simulink model "SimulinkSampleMotorWheelMode_R2017a"  (R2019a)
settings: Solver=VariableStepAuto  StartTime=0.0  StopTime=10.0  RelTol=1e-3
libraries: instrumentlib x3
settings Model: Creator=go_71  LastModifiedBy=Eureka Dynamics
settings DebuggingCC: UnconnectedInputMsg=none  UnconnectedOutputMsg=none  UnconnectedLineMsg=none  ArithmeticOperatorsInVariantConditions=warning
settings ModelReferenceCC: EnableRefExpFcnMdlSchedulingChecks=off
settings RTWCC: Description=Generic Real-Time Target
settings CodeAppCC: StateflowObjectComments=on

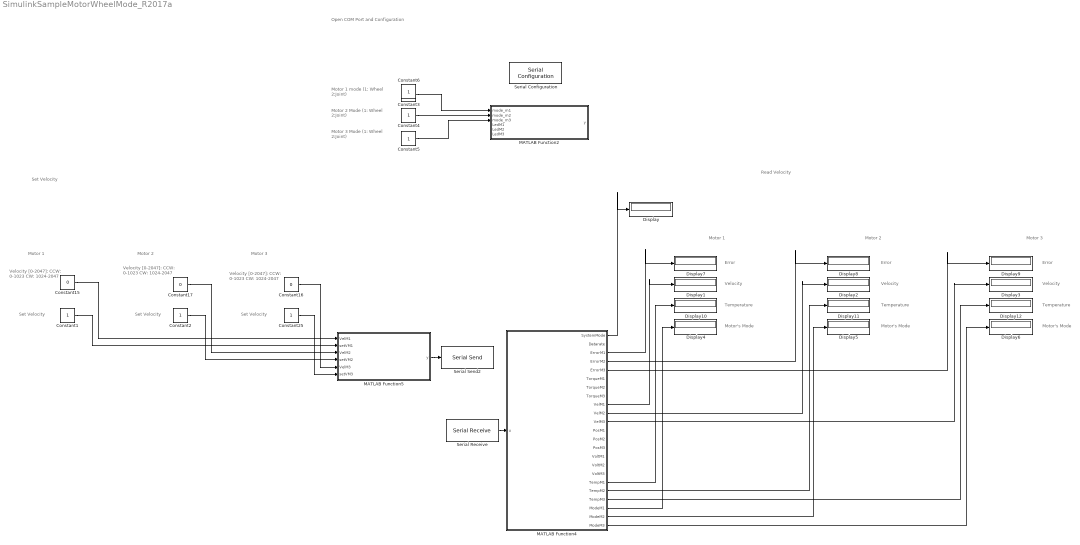
== system SimulinkSampleMotorWheelMode_R2017a ==
  note: Open COM Port and Configuration
  note: Motor's Mode
  note: Motor 3
  note: Temperature
  note: Error
  note: Temperature
  note: Error
  note: Velocity
  note: Velocity
  note: Motor's Mode
  note: Motor's Mode
  note: Error
  note: Temperature
  note: Velocity
  note: Motor 1
  note: Motor 2
  note: Motor 1 mode
      | (1: Wheel 2:Joint)
  note: Motor 2 Mode
      | (1: Wheel 2:Joint)
  note: Motor 3 Mode
      | (1: Wheel 2:Joint)
  note: Motor 1
  note: Motor 2
  note: Motor 3
  note: Read Velocity
  note: Set Velocity
  note: Velocity
      | [0-2047]:
      | CCW: 0-1023
      | CW: 1024-2047
  note: Set Velocity
  note: Set Velocity
  note: Velocity
      | [0-2047]:
      | CCW: 0-1023
      | CW: 1024-2047
  note: Set Velocity
  note: Velocity
      | [0-2047]:
      | CCW: 0-1023
      | CW: 1024-2047
  Constant{1..6,25} (7 alike) : Constant  SampleTime=1
  Constant15 : Constant  Value=0  SampleTime=1
  Constant16 : Constant  Value=0  SampleTime=1
  Constant17 : Constant  Value=0  SampleTime=1
  Display{,1..12} (13 alike) : Display
  MATLAB Function2 : MATLAB Function  Priority=1  TreatAsAtomicUnit=on  SystemSampleTime=1
  MATLAB Function4 : MATLAB Function  Priority=3  TreatAsAtomicUnit=on
  MATLAB Function5 : MATLAB Function  Priority=2  TreatAsAtomicUnit=on
  Serial Configuration : instrumentlib/Serial Configuration  Priority=-200000  ComPortMenu=<Please select a port...>  ComPort=<Please select a port...>  BaudRate=9600  DataBits=8  Parity=none  StopBits=1  FlowControl=none  Timeout=10  ByteOrder=LittleEndian
  Serial Receive : instrumentlib/Serial Receive  ComPortMenu=<Please select a port...>  ComPort=<Please select a port...>  DataSize="[32   1]"  DataType=uint8  EnableBlockingMode=on  ActionDataUnavailable=Output last received value  CustomValue=0  SampleTime=0.01
  Serial Send2 : instrumentlib/Serial Send  ComPortMenu=<Please select a port...>  ComPort=<Please select a port...>  Terminator=<none>  EnableBlockingMode=on
  wires:
  Constant3/1 -> MATLAB Function2/1(mode_m1)
  Constant5/1 -> MATLAB Function2/3(mode_m3)
  Constant25/1 -> MATLAB Function5/6(setVM3)
  Constant4/1 -> MATLAB Function2/2(mode_m2)
  Constant1/1 -> MATLAB Function5/2(setVM1)
  Constant2/1 -> MATLAB Function5/4(setVM2)
  Constant15/1 -> MATLAB Function5/1(VelM1)
  Constant17/1 -> MATLAB Function5/3(VelM2)
  Constant16/1 -> MATLAB Function5/5(VelM3)
  MATLAB Function4/22(ModeM2) -> Display5/1
  MATLAB Function4/21(ModeM1) -> Display4/1
  MATLAB Function4/20(TempM3) -> Display12/1
  MATLAB Function4/4(ErrorM2) -> Display8/1
  MATLAB Function4/19(TempM2) -> Display11/1
  MATLAB Function4/3(ErrorM1) -> Display7/1
  MATLAB Function4/1(SystemMode) -> Display/1
  Serial Receive/1 -> MATLAB Function4/1(u)
  MATLAB Function4/18(TempM1) -> Display10/1
  MATLAB Function4/5(ErrorM3) -> Display9/1
  MATLAB Function4/23(ModeM3) -> Display6/1
  MATLAB Function4/9(VelM1) -> Display1/1
  MATLAB Function4/10(VelM2) -> Display2/1
  MATLAB Function4/11(VelM3) -> Display3/1
  MATLAB Function5/1(y) -> Serial Send2/1

== matlab function SimulinkSampleMotorWheelMode_R2017a/MATLAB Function2 ==
  data: y output; mode_m1 input; mode_m2 input; mode_m3 input; LedM1 input; LedM2 input; LedM3 input
function y  = setMotorsConfiguration(mode_m1,mode_m2,mode_m3,LedM1,LedM2,LedM3)
% Motor Configuration Packet

% mode_m1=1 -> Wheel
% mode_m1=2 -> Joint

s.init          = 122;
s.mode          = 3;      % 3=motor configuration
s.set_mode_m1   = 48 ;    % 48 = char '0' 49 = char '1'
s.set_mode_m2   = 48 ;    % 48 = char '0' 49 = char '1'
s.set_mode_m3   = 48 ;    % 48 = char '0' 49 = char '1'
s.mode_m1       = 49 ;  %49 = char '1' Wheel   50 = char '2' Joint
s.mode_m2       = 49 ;  %49 = char '1' Wheel   50 = char '2' Joint
s.mode_m3       = 49 ;  %49 = char '1' Wheel   50 = char '2' Joint

if mode_m1~=0
    s.set_mode_m1 = 49 ;  
    if mode_m1==1 %Mode Wheel
        s.mode_m1 = 49 ;
    elseif mode_m1==2  
        s.mode_m1 = 50 ;  
    end
end

if mode_m2~=0
    s.set_mode_m2 = 49 ;   
    if mode_m2==1 % Mode Wheel
        s.mode_m2 = 49 ; 
    elseif mode_m2==2  
        s.mode_m2 = 50 ;
    end
end

if mode_m3~=0
    s.set_mode_m3 = 49 ; 
    if mode_m3 == 1 % Mode Wheel
        s.mode_m3 = 49 ; 
    elseif mode_m3==2  
        s.mode_m3 = 50 ;
    end
end


s.set_id_m1 = 0 ;
s.set_id_m2 = 0 ;
s.set_id_m3 = 0 ;

s.id_m1 = 0;
s.id_m2 = 0;
s.id_m3 = 0;

LEDM1 = 48;
if LedM1 ==1
    LEDM1 =49;
end

LEDM2 = 48;
if LedM2 ==1
    LEDM2 =49;
end

LEDM3 = 48;
if LedM3 ==1
    LEDM3 =49;
end

s.turnon_led_m1 = LEDM1;  %48:0  49:1
s.turnon_led_m2 = LEDM2;
s.turnon_led_m3 = LEDM3;
s.not_used17 = 0;
s.not_used18 = 0;
s.not_used19 = 0;
s.not_used20 = 0;
s.not_used21 = 0;
s.not_used22 = 0;
s.not_used23 = 0;
s.not_used24 = 0;
s.not_used25 = 0;
s.not_used26 = 0;
s.not_used27 = 0;
s.not_used28 = 0;
s.not_used29 = 0;
s.not_used30 = 1;  %Thiss byte has to be 1. 
s.finish = 123;

ArrToSend = uint8([s.init ;s.mode ; s.set_mode_m1; s.set_mode_m2; s.set_mode_m3; s.mode_m1;s.mode_m2;s.mode_m3;s.set_id_m1;s.set_id_m2;s.set_id_m3;s.id_m1;s.id_m2;s.id_m3;s.turnon_led_m1;s.turnon_led_m2;s.turnon_led_m3;s.not_used17;s.not_used18;s.not_used19;s.not_used20;s.not_used21;s.not_used22;s.not_used23;s.not_used24;s.not_used25;s.not_used26;s.not_used27;s.not_used28;s.not_used29; s.not_used30;s.finish]);

y = ArrToSend;

== matlab function SimulinkSampleMotorWheelMode_R2017a/MATLAB Function4 ==
  data: u input; SystemMode output; Datarate output; ErrorM1 output; ErrorM2 output; ErrorM3 output; TorqueM1 output double size=[16 1]; TorqueM2 output; TorqueM3 output; VelM1 output; VelM2 output; VelM3 output; PosM1 output; PosM2 output; PosM3 output; VoltM1 output; VoltM2 output; VoltM3 output; TempM1 output; TempM2 output; TempM3 output; ModeM1 output; ModeM2 output; ModeM3 output
function  [SystemMode,Datarate,ErrorM1,ErrorM2,ErrorM3,TorqueM1,TorqueM2,TorqueM3,VelM1,VelM2,VelM3,PosM1,PosM2,PosM3,VoltM1,VoltM2,VoltM3,TempM1,TempM2,TempM3, ModeM1,ModeM2,ModeM3] = ReadMotorsPacket(u)
%Read Motor Paquet
coder.extrinsic('extractBetween'); 
coder.extrinsic('str2num'); 

SystemMode = 0;
Datarate=0;
ErrorM1=0;
ErrorM2=0;
ErrorM3=0;
TorqueM1 = 0;
TorqueM2=0;
TorqueM3=0;
VelM1=0;
VelM2=0;
VelM3=0;
PosM1=0;
PosM2=0;
PosM3=0;
VoltM1=0;
VoltM2=0;
VoltM3=0;
TempM1=0;
TempM2=0;
TempM3=0;
ModeM1=0;
ModeM2=0;
ModeM3=0;

Utest = char(u);

SystemMode = double(uint8(u(2,1)));   %1:Motor   2:Encoder
Datarate = double(uint8(u(3,1))); %0:Default 100 ms

ErrorM1=double(uint8(u(4,1)));
ErrorM2=double(uint8(u(5,1)));
ErrorM3=double(uint8(u(6,1)));

TorqueM1Aux = (typecast([uint8(u(7,1)) uint8(u(8,1))],'uint16'));
TorqueM2Aux = (typecast([uint8(u(9,1)) uint8(u(10,1))],'uint16'));
TorqueM3Aux = (typecast([uint8(u(11,1)) uint8(u(12,1))],'uint16'));

TorqueM1 =  double(bitand(TorqueM1Aux,uint16(1023)))*0.1;
TorqueM2 = double(bitand(TorqueM2Aux,uint16(1023)))*0.1;
TorqueM3 = double(bitand(TorqueM3Aux,uint16(1023)))*0.1;

VelM1Aux = typecast([uint8(u(13,1)) uint8(u(14,1))],'uint16');
VelM2Aux = typecast([uint8(u(15,1)) uint8(u(16,1))],'uint16');
VelM3Aux = typecast([uint8(u(17,1)) uint8(u(18,1))],'uint16');
VelM1 = double(bitand(VelM1Aux,uint16(1023)))*0.1;
VelM2 = double(bitand(VelM2Aux,uint16(1023)))*0.1;
VelM3 = double(bitand(VelM3Aux,uint16(1023)))*0.1;

PosM1Aux = typecast([uint8(u(19,1)) uint8(u(20,1))],'uint16');
PosM2Aux = typecast([uint8(u(21,1)) uint8(u(22,1))],'uint16');
PosM3Aux = typecast([uint8(u(23,1)) uint8(u(24,1))],'uint16');
PosM1 = double(PosM1Aux);%*0.29;
PosM2 = double(PosM2Aux);%*0.29;
PosM3 = double(PosM3Aux);%*0.29;

VoltM1 = double(uint8(u(25,1)))/10.0;
VoltM2 = double(uint8(u(26,1)))/10.0;
VoltM3 = double(uint8(u(27,1)))/10.0;

TempM1 = double(uint8(u(28,1)));
TempM2 = double(uint8(u(29,1)));
TempM3 = double(uint8(u(30,1)));

Mode  = de2bi(double(uint8(u(31,1))));
sm = size(Mode,2);
dif = 6-sm;
Mode6bits=[0 0 0 0 0 0 ];
for i=1:sm
    Mode6bits(i) = Mode(i);
end
for d=1:dif
    Mode6bits(sm+d)=0;
end

ModeM1Aux = binaryToDecimal(Mode6bits(1:2),'LSB');  %2017
ModeM2Aux = binaryToDecimal(Mode6bits(3:4),'LSB');  %2017
ModeM3Aux = binaryToDecimal(Mode6bits(5:6),'LSB');  %2017

% ModeM1Aux = bi2de(Mode6bits(1:2));
% ModeM2Aux = bi2de(Mode6bits(3:4));
% ModeM3Aux = bi2de(Mode6bits(5:6));

ModeM1 = double(ModeM1Aux); %1:Wheel 2:Joint
ModeM2 = double(ModeM2Aux);%1:Wheel 2:Joint
ModeM3 = double(ModeM3Aux);%1:Wheel 2:Joint

nop=1;

== matlab function SimulinkSampleMotorWheelMode_R2017a/MATLAB Function5 ==
  data: VelM1 input; setVM1 input; y output; VelM2 input; setVM2 input; VelM3 input; setVM3 input
function y = setMotorsVelocity(VelM1,setVM1,VelM2,setVM2,VelM3,setVM3)

% Write Motor Packet
coder.extrinsic('num2str'); 
Arr = uint8([1:32]);

setV3   = bitshift(setVM3,2); 
setV2   = bitshift(setVM2,1); 
setV1   = setVM1;
setVaux = bitor(setV3,setV2);
setV    = bitor(setV1,setVaux);

inp         = de2bi(VelM1,16);
LBits_arr   = inp(1,1:8);
HBits_arr   = inp(1,9:16);
% LBitsM1     = bi2de(LBits_arr);
% HBitsM1     = bi2de(HBits_arr);
LBitsM1 = binaryToDecimal(LBits_arr,'LSB');  %2017
HBitsM1 = binaryToDecimal(HBits_arr,'LSB');  %2017

inp2        = de2bi(VelM2,16);
LBits_arr2  = inp2(1,1:8);
HBits_arr2  = inp2(1,9:16);
% LBitsM2     = bi2de(LBits_arr2);
% HBitsM2     = bi2de(HBits_arr2);
LBitsM2 = binaryToDecimal(LBits_arr2,'LSB');  %2017
HBitsM2 = binaryToDecimal(HBits_arr2,'LSB');  %2017

inp3        = de2bi(VelM3,16);
LBits_arr3  = inp3(1,1:8);
HBits_arr3  = inp3(1,9:16);
% LBitsM3     = bi2de(LBits_arr3);
% HBitsM3     = bi2de(HBits_arr3);
LBitsM3 = binaryToDecimal(LBits_arr3,'LSB');  %2017
HBitsM3 = binaryToDecimal(HBits_arr3,'LSB');  %2017

Arr(1,1) =  122;
Arr(1,2) =  2;
Arr(1,3) =  0; %SET ANGLE LIMIT   0:0° 512:150°  a 1023:300°
Arr(1,4) =  0; %CW M1
Arr(1,5) =  0; %CW M1
Arr(1,6) =  0; %CW M2
Arr(1,7) =  0; %CW M2
Arr(1,8) =  0; %CW M3 
Arr(1,9) =  0; %CW M3
Arr(1,10) =  0; %CCW M1
Arr(1,11) =  0; %CCW M1
Arr(1,12) =  0; %CCW M2
Arr(1,13) =  0; %CCW M2
Arr(1,14) =  0; %CCW M3
Arr(1,15) =  0; %CCW M3
Arr(1,16) = setV; %SET MOVING SPEED
Arr(1,17) =  LBitsM1;
Arr(1,18) =  HBitsM1;
Arr(1,19) =  LBitsM2;
Arr(1,20) =  HBitsM2;
Arr(1,21) =  LBitsM3;
Arr(1,22) =  HBitsM3;
Arr(1,23) =  0; %SET POSITION
Arr(1,24) =  0;
Arr(1,25) =  0;
Arr(1,26) =  0;
Arr(1,27) =  0;
Arr(1,28) =  0;
Arr(1,29) =  0;
Arr(1,30) =  0;
Arr(1,31) =  0;
Arr(1,32) =  123;

y = Arr;
